simulink model "Lab4ControlSystems"  (R2015a)
settings: Solver=ode23t  StartTime=0.0  StopTime=4  RelTol=1e-3
libraries: dspsrcs4 x1
settings Model: Creator=Quswar Mahmood Abid  LastModifiedBy=Quswar Mahmood Abid

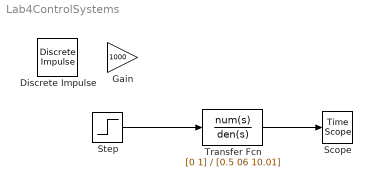
== system Lab4ControlSystems ==
  Discrete Impulse : dspsrcs4/Discrete  Impulse  Delay=0  SampleTime=.001  FrameSample=1  dataType=double  isSigned=on  wordLen=16  udDataType=sfix(16)  fracBitsMode=Best precision  numFracBits=15  OutDataTypeStr=double  LastOutDataTypeStr=double
  Gain : Gain  Gain=1000
  Scope : TimeScope
  Step : Step  Time=0  SampleTime=0
  Transfer Fcn : TransferFcn  Numerator=[0 1]  Denominator=[0.5 06 10.01]
  wires:
  Transfer Fcn/1 -> Scope/1
  Step/1 -> Transfer Fcn/1
